simulink model "robotMobilny"  (Simulink 9.1)
settings: Solver=ode45  StartTime=0.0  StopTime=9.2  MaxStep=0.01  RelTol=1e-3
values from neighbouring files (symbols this model uses):
  B = 1    [GSR_trajectory.m]    (also in init.m = [b/(r*ng) -b/(r*ng); 1/(r*ng) 1/(r*ng)])
  H = [((2*b^2)/(r^2))*(Ksi+1/(ng^2)*Ksi_m) 0;0 (2/(r^2))*(Ksi+1/(ng^2)*Ksi_m)]    [init.m]
  J_inv = inv(J)    [init.m]
  K_m = [km 0; 0 km]    [init.m]
  kc = ki + 50    (= 109.789741582)    [init.m]
  ki = (T*om_0^2)/(K*kp)    (= 59.7897415818)    [init.m]
  kp = (2*T*zeta_0*om_0-1)/K    (= 2.17361702128)    [init.m]
  M_inv = inv(M)    [init.m]
  N_inv = inv(N)    [init.m]
  omega_dc = [80;80]    [init.m]
  R_m_inv = inv(R_m)    [init.m]
  Tf = 1/ki    (= 0.016725277172)    [init.m]
  Um = [9;9]    [init.m]
  Umax = 9    [init.m]
settings Model: Creator=hp  LastModifiedBy=hp
settings DataIOCC: SaveFormat=Dataset
settings OptimizationCC: LifeSpan=auto
settings DebuggingCC: UnderspecifiedInitializationDetection=Simplified  MergeDetectMultiDrivingBlocksExec=error  SFUnexpectedBacktrackingDiag=error  SFNoUnconditionalDefaultTransitionDiag=error  SFExecutionAtInitializationDiag=warning
settings HardwareCC: ProdBitPerPointer=64  ProdBitPerSizeT=64  ProdBitPerPtrDiffT=64  ProdLargestAtomicFloat=Float  ProdIntDivRoundTo=Zero  ProdEndianess=LittleEndian  ProdWordSize=64  ProdHWDeviceType=Intel->x86-64 (Windows64)
settings ModelReferenceCC: PropagateSignalLabelsOutOfModel=on
settings CodeAppCC: StateflowObjectComments=off
settings GRTTargetCC: TargetLangStandard=C99 (ISO)  CombineOutputUpdateFcns=on  GRTInterface=off
settings ConfigComp: CovMetricSettings=dwe  CovHtmlReporting=off  CovSaveCumulativeToWorkspaceVar=off  CovSaveSingleToWorkspaceVar=off  CovExternalEMLEnable=on

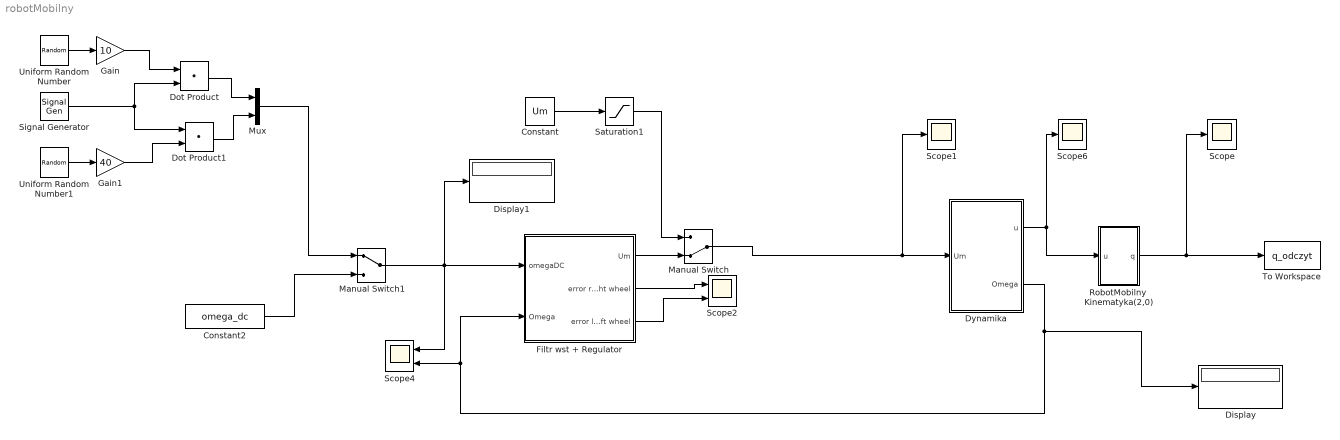
== system robotMobilny ==
  Constant : Constant  Value=Um
  Constant2 : Constant  Value=omega_dc
  Display : Display
  Display1 : Display
  Dot Product : DotProduct  InputSameDT=on  OutDataTypeStr=Inherit: Inherit via internal rule
  Dot Product1 : DotProduct  InputSameDT=on  OutDataTypeStr=Inherit: Inherit via internal rule
  Dynamika : Subsystem
  Filtr wst + Regulator : Subsystem
  Gain : Gain  Gain=10
  Gain1 : Gain  Gain=40
  Manual Switch : ManualSwitch  CurrentSetting=0
  Manual Switch1 : ManualSwitch
  Mux : Mux  Inputs=2
  RobotMobilny  Kinematyka(2,0) : Subsystem
  Saturation1 : Saturate  UpperLimit=Umax  LowerLimit=-Umax
  Scope : Scope
  Scope1 : Scope
  Scope2 : Scope  NumInputPorts=2
  Scope4 : Scope  NumInputPorts=2
  Scope6 : Scope
  Signal Generator : SignalGenerator  WaveForm=square  Units=rad/sec
  To Workspace : ToWorkspace  VariableName=q_odczyt  SaveFormat=Structure With Time  SampleTime=-1
  Uniform Random Number : UniformRandomNumber  SampleTime=1
  Uniform Random Number1 : UniformRandomNumber  SampleTime=1
  wires:
  RobotMobilny  Kinematyka(2,0)/1(q) -> To Workspace/1, Scope/1
  Dynamika/1(u) -> Scope6/1, RobotMobilny  Kinematyka(2,0)/1(u)
  Manual Switch/1 -> Scope1/1, Dynamika/1("Um ")
  Constant/1 -> Saturation1/1
  Dynamika/2(Omega) -> Scope4/2, Filtr wst + Regulator/2(Omega), Display/1
  Filtr wst + Regulator/1(Um) -> Manual Switch/2
  Filtr wst + Regulator/2(error right wheel) -> Scope2/1
  Filtr wst + Regulator/3(error left wheel) -> Scope2/2
  Saturation1/1 -> Manual Switch/1
  Manual Switch1/1 -> Display1/1, Scope4/1, Filtr wst + Regulator/1(omegaDC)
  Constant2/1 -> Manual Switch1/2
  Uniform Random Number/1 -> Gain/1
  Signal Generator/1 -> Dot Product1/1, Dot Product/2
  Uniform Random Number1/1 -> Gain1/1
  Dot Product/1 -> Mux/1
  Dot Product1/1 -> Mux/2
  Mux/1 -> Manual Switch1/1
  Gain/1 -> Dot Product/1
  Gain1/1 -> Dot Product1/2

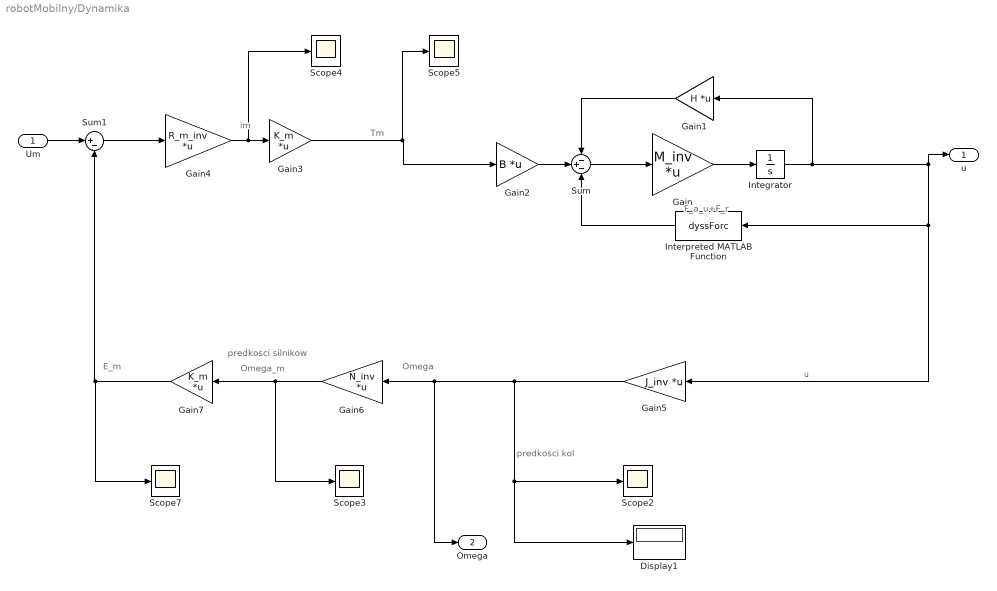
== system robotMobilny/Dynamika ==
  note: predkosci silnikow
  note: predkosci kol
  note: E_m
  note: Omega_m
  note: Omega
  note: im
  note: Tm
  note: F_a_u+F_r
  "Um " : Inport
  Display1 : Display
      settings: Decimation=2
  Gain : Gain  Gain=M_inv  Multiplication=Matrix(K*u)
  Gain1 : Gain  Gain=H  Multiplication=Matrix(K*u)
  Gain2 : Gain  Gain=B  Multiplication=Matrix(K*u)
  Gain3 : Gain  Gain=K_m  Multiplication=Matrix(K*u)
  Gain4 : Gain  Gain=R_m_inv  Multiplication=Matrix(K*u)
  Gain5 : Gain  Gain=J_inv  Multiplication=Matrix(K*u)
  Gain6 : Gain  Gain=N_inv  Multiplication=Matrix(K*u)
  Gain7 : Gain  Gain=K_m  Multiplication=Matrix(K*u)
  Integrator : Integrator  InitialCondition=[0;0]
  Interpreted MATLAB Function : MATLABFcn  MATLABFcn=dyssForc
  Scope{2..5,7} (5 alike) : Scope
  Sum : Sum  Inputs=-+-
  Sum1 : Sum  Inputs=|+-
  u : Outport
  Omega : Outport  Port=2
  wires:
  Gain7/1 -> Scope7/1, Sum1/2
  Gain6/1 -> Scope3/1, Gain7/1
  Gain5/1 -> Scope2/1, Display1/1, Omega/1, Gain6/1
  Gain1/1 -> Sum/1
  Sum1/1 -> Gain4/1
  Gain4/1 -> Scope4/1, Gain3/1
  Interpreted MATLAB Function/1 -> Sum/3
  Integrator/1 -> u/1, Gain5/1, Interpreted MATLAB Function/1, Gain1/1  "u"
  Gain3/1 -> Scope5/1, Gain2/1
  Gain2/1 -> Sum/2
  Sum/1 -> Gain/1
  Gain/1 -> Integrator/1
  "Um "/1 -> Sum1/1

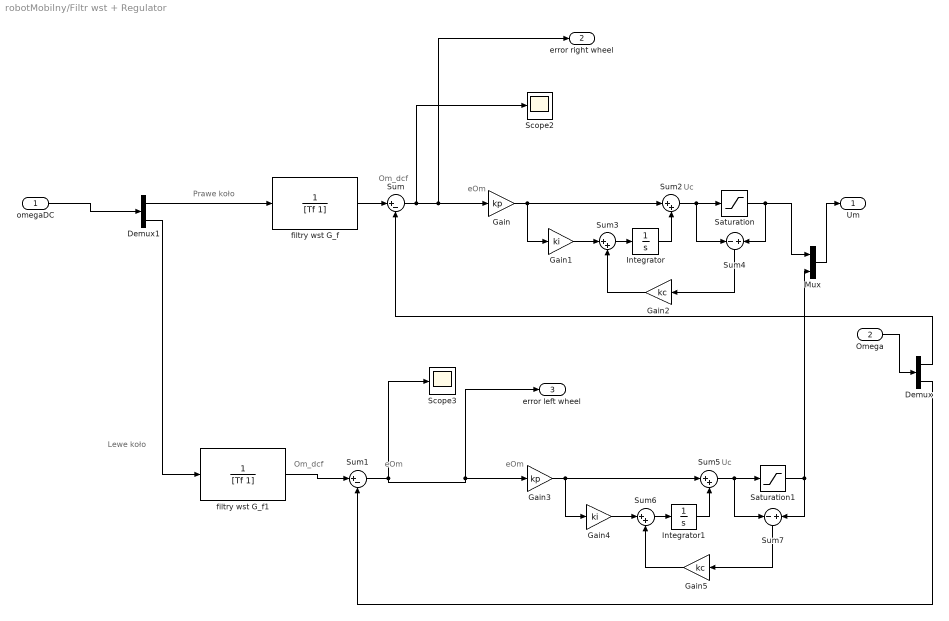
== system robotMobilny/Filtr wst + Regulator ==
  note: Uc
  note: Prawe koło
  note: Om_dcf
  note: eOm
  note: Om_dcf
  note: eOm
  note: Lewe koło
  note: eOm
  note: Uc
  omegaDC : Inport
  Omega : Inport  Port=2
  Demux : Demux  Outputs=2
  Demux1 : Demux  Outputs=2
  Gain : Gain  Gain=kp
  Gain1 : Gain  Gain=ki
  Gain2 : Gain  Gain=kc
  Gain3 : Gain  Gain=kp
  Gain4 : Gain  Gain=ki
  Gain5 : Gain  Gain=kc
  Integrator : Integrator
  Integrator1 : Integrator
  Mux : Mux  Inputs=2
  Saturation : Saturate  UpperLimit=Umax  LowerLimit=-Umax
  Saturation1 : Saturate  UpperLimit=Umax  LowerLimit=-Umax
  Scope2 : Scope
  Scope3 : Scope
  Sum : Sum  Inputs=|+-
  Sum1 : Sum  Inputs=|+-
  Sum{2..3,5..6} (4 alike) : Sum  Inputs=|++
  Sum4 : Sum  Inputs=-+
  Sum7 : Sum  Inputs=-+
  filtry wst G_f : TransferFcn  Denominator=[Tf 1]
  filtry wst G_f1 : TransferFcn  Denominator=[Tf 1]
  Um : Outport
  error right wheel : Outport  Port=2
  error left wheel : Outport  Port=3
  wires:
  filtry wst G_f/1 -> Sum/1
  Sum/1 -> Gain/1, error right wheel/1, Scope2/1
  Demux1/1 -> filtry wst G_f/1
  Demux1/2 -> filtry wst G_f1/1
  Demux/2 -> Sum1/2
  Saturation/1 -> Sum4/2, Mux/1
  filtry wst G_f1/1 -> Sum1/1
  Demux/1 -> Sum/2
  Saturation1/1 -> Mux/2, Sum7/2
  Mux/1 -> Um/1
  Omega/1 -> Demux/1
  omegaDC/1 -> Demux1/1
  Gain/1 -> Gain1/1, Sum2/1
  Gain1/1 -> Sum3/1
  Sum3/1 -> Integrator/1
  Sum2/1 -> Sum4/1, Saturation/1
  Integrator/1 -> Sum2/2
  Sum4/1 -> Gain2/1
  Gain2/1 -> Sum3/2
  Sum6/1 -> Integrator1/1
  Sum1/1 -> error left wheel/1, Gain3/1, Scope3/1
  Gain3/1 -> Gain4/1, Sum5/1
  Gain5/1 -> Sum6/2
  Sum7/1 -> Gain5/1
  Sum5/1 -> Sum7/1, Saturation1/1
  Gain4/1 -> Sum6/1
  Integrator1/1 -> Sum5/2

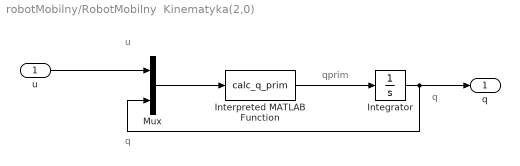
== system robotMobilny/RobotMobilny  Kinematyka(2,0) ==
  note: qprim
  note: q
  note: u
  note: q
  u : Inport
  Integrator : Integrator  InitialCondition=[0; 0; 0]
  Interpreted MATLAB Function : MATLABFcn  MATLABFcn=calc_q_prim  OutputDimensions=3
  Mux : Mux  Inputs=2
  q : Outport
  wires:
  Interpreted MATLAB Function/1 -> Integrator/1
  Integrator/1 -> q/1, Mux/2
  Mux/1 -> Interpreted MATLAB Function/1
  u/1 -> Mux/1
